simulink model "Lab3Simulink"  (R2024b)
settings: Solver=FixedStepAuto  StartTime=0.0  StopTime=inf  FixedStep=0.01  RelTol=1e-3  EnableMultiTasking=on
libraries: stm32f4xxblockslib x9, simulink x3, stm32g4xxblockslib x3
settings Model: STM32="{\"EncoderBlockForG4\":[{\"ID\":\"Lab3Simulink:156\"},{\"ID\":\"Lab3Simulink:162\"},{\"ID\":\"Lab3Simulink:166\"}],\"DigitalPortRead\":[{\"ID\":\"Lab3Simulink:9\"},{\"ID\":\"Lab3Simulink:11\"},{\"ID\":\"Lab3Simulink:112\"},{\"ID\":\"Lab3Simulink:113\"},{\"ID\":\"Lab3Simulink:119\"},{\"ID\":\"Lab3Simulink:120\"},{\"ID\":\"Lab3Simulink:198\"},{\"ID\":\"Lab3Simulink:199\"},{\"ID\":\"Lab3Simulink:200\"}]}"  Creator=lenovo  LastModifiedBy=lenovo
settings OptimizationCC: DefaultParameterBehavior=Inlined  EnhancedBackFolding=on  PassReuseOutputArgsAs=Individual arguments  ZeroExternalMemoryAtStartup=off  ZeroInternalMemoryAtStartup=off  MaxStackSize=512  OptimizeBlockOrder=speed  DifferentSizesBufferReuse=on  OptimizationCustomize=off  EfficientTunableParamExpr=on
settings DebuggingCC: ParameterTunabilityLossMsg=error
settings HardwareCC: ProdBitPerPointer=32  ProdBitPerSizeT=32  ProdBitPerPtrDiffT=32  ProdLargestAtomicInteger=Long  ProdLargestAtomicFloat=Double  ProdWordSize=32  ProdLongLongMode=on  ProdHWDeviceType=ARM Compatible->ARM Cortex-M
settings SFSimCC: MATLABDynamicMemAlloc=off
settings RTWCC: Description=Embedded Coder  SystemTargetFile=ert.tlc  HardwareBoard=STM32G4xx Based  TemplateMakefile=ert_default_tmf  Toolchain=GNU Tools for ARM Embedded Processors
settings CodeAppCC: ForceParamTrailComments=on  IgnoreCustomStorageClasses=off  OperatorAnnotations=on  SimulinkDataObjDesc=on  SFDataObjDesc=on  InsertBlockDesc=on
settings ERTTargetCC: TargetLangStandard=C99 (ISO)  CodeReplacementLibrary=ARM Cortex-M  ExtModeTransport=3  ExtModeStaticAlloc=on  ExtModeStaticAllocSize=2048  ExtModeMexFile=ext_xcp  ExtModeIntrfLevel=Level2 - Open

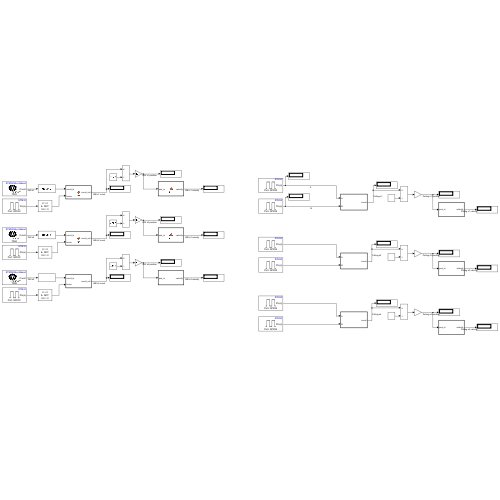
[thumbnail: Simulink's stored preview of the top-level diagram]
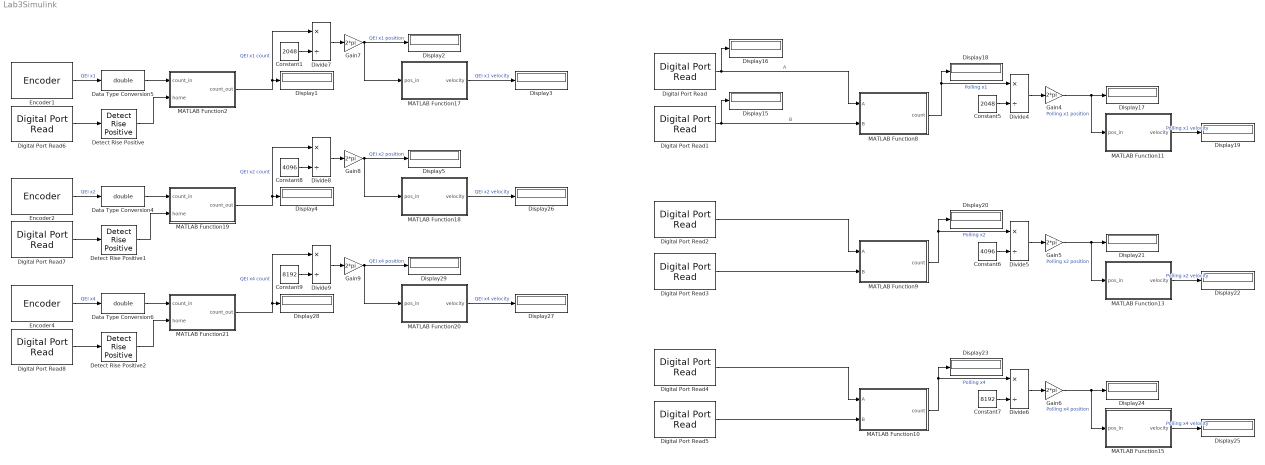
== system Lab3Simulink ==
  Constant1 : Constant  Value=2048
  Constant5 : Constant  Value=2048
  Constant6 : Constant  Value=4096
  Constant7 : Constant  Value=8192
  Constant8 : Constant  Value=4096
  Constant9 : Constant  Value=8192
  Data Type Conversion4 : DataTypeConversion  OutDataTypeStr=double  SaturateOnIntegerOverflow=off  RndMeth=Floor
  Data Type Conversion5 : DataTypeConversion  OutDataTypeStr=double  SaturateOnIntegerOverflow=off  RndMeth=Floor
  Data Type Conversion6 : DataTypeConversion  OutDataTypeStr=double  SaturateOnIntegerOverflow=off  RndMeth=Floor
  Detect Rise Positive : simulink/Logic and Bit Operations/Detect Rise Positive  vinit=0  OutDataTypeStr=boolean
  Detect Rise Positive1 : simulink/Logic and Bit Operations/Detect Rise Positive  vinit=0  OutDataTypeStr=boolean
  Detect Rise Positive2 : simulink/Logic and Bit Operations/Detect Rise Positive  vinit=0  OutDataTypeStr=boolean
  Digital Port Read : stm32f4xxblockslib/Digital Port Read  PortName=GPIOB  PinNumber=[4]  ReadOperation=on  IOAsArray=on  SampleTime=-1  EnableSimPort=off  hoistedMaskSrc=ECSoC/ECSimCodegen/Digital Port Read
      settings: LibrarySourceBlock=stm32g4xxblockslib/Digital Port Read
  Digital Port Read1 : stm32f4xxblockslib/Digital Port Read  PortName=GPIOB  PinNumber=[5]  ReadOperation=on  IOAsArray=on  SampleTime=-1  EnableSimPort=off  hoistedMaskSrc=ECSoC/ECSimCodegen/Digital Port Read
      settings: LibrarySourceBlock=stm32g4xxblockslib/Digital Port Read
  Digital Port Read2 : stm32f4xxblockslib/Digital Port Read  PortName=GPIOB  PinNumber=[4]  ReadOperation=on  IOAsArray=on  SampleTime=-1  EnableSimPort=off  hoistedMaskSrc=ECSoC/ECSimCodegen/Digital Port Read
      settings: LibrarySourceBlock=stm32g4xxblockslib/Digital Port Read
  Digital Port Read3 : stm32f4xxblockslib/Digital Port Read  PortName=GPIOB  PinNumber=[5]  ReadOperation=on  IOAsArray=on  SampleTime=-1  EnableSimPort=off  hoistedMaskSrc=ECSoC/ECSimCodegen/Digital Port Read
      settings: LibrarySourceBlock=stm32g4xxblockslib/Digital Port Read
  Digital Port Read4 : stm32f4xxblockslib/Digital Port Read  PortName=GPIOB  PinNumber=[4]  ReadOperation=on  IOAsArray=on  SampleTime=-1  EnableSimPort=off  hoistedMaskSrc=ECSoC/ECSimCodegen/Digital Port Read
      settings: LibrarySourceBlock=stm32g4xxblockslib/Digital Port Read
  Digital Port Read5 : stm32f4xxblockslib/Digital Port Read  PortName=GPIOB  PinNumber=[5]  ReadOperation=on  IOAsArray=on  SampleTime=-1  EnableSimPort=off  hoistedMaskSrc=ECSoC/ECSimCodegen/Digital Port Read
      settings: LibrarySourceBlock=stm32g4xxblockslib/Digital Port Read
  Digital Port Read6 : stm32f4xxblockslib/Digital Port Read  PortName=GPIOC  PinNumber=[13]  ReadOperation=on  IOAsArray=on  SampleTime=-1  EnableSimPort=off  hoistedMaskSrc=ECSoC/ECSimCodegen/Digital Port Read
      settings: LibrarySourceBlock=stm32g4xxblockslib/Digital Port Read
  Digital Port Read7 : stm32f4xxblockslib/Digital Port Read  PortName=GPIOC  PinNumber=[13]  ReadOperation=on  IOAsArray=on  SampleTime=-1  EnableSimPort=off  hoistedMaskSrc=ECSoC/ECSimCodegen/Digital Port Read
      settings: LibrarySourceBlock=stm32g4xxblockslib/Digital Port Read
  Digital Port Read8 : stm32f4xxblockslib/Digital Port Read  PortName=GPIOC  PinNumber=[13]  ReadOperation=on  IOAsArray=on  SampleTime=-1  EnableSimPort=off  hoistedMaskSrc=ECSoC/ECSimCodegen/Digital Port Read
      settings: LibrarySourceBlock=stm32g4xxblockslib/Digital Port Read
  Display{1..5,15..29} (20 alike) : Display
  Divide{4..9} (6 alike) : Product  Inputs=*/
  Encoder1 : stm32g4xxblockslib/Encoder  TimerModule=TIM3  EnableResetInput=off  OutputCountAfterFirstIndex=off  OutputValidIndex=off  OutputDirection=off  OutputStatus=off  SampleTime=-1
  Encoder2 : stm32g4xxblockslib/Encoder  TimerModule=TIM4  EnableResetInput=off  OutputCountAfterFirstIndex=off  OutputValidIndex=off  OutputDirection=off  OutputStatus=off  SampleTime=-1
  Encoder4 : stm32g4xxblockslib/Encoder  TimerModule=TIM8  EnableResetInput=off  OutputCountAfterFirstIndex=off  OutputValidIndex=off  OutputDirection=off  OutputStatus=off  SampleTime=-1
  Gain{4..9} (6 alike) : Gain  Gain=2*pi
  MATLAB Function10 : MATLAB Function  TreatAsAtomicUnit=on
  MATLAB Function11 : MATLAB Function  TreatAsAtomicUnit=on
  MATLAB Function13 : MATLAB Function  TreatAsAtomicUnit=on
  MATLAB Function15 : MATLAB Function  TreatAsAtomicUnit=on
  MATLAB Function17 : MATLAB Function  TreatAsAtomicUnit=on
  MATLAB Function18 : MATLAB Function  TreatAsAtomicUnit=on
  MATLAB Function19 : MATLAB Function  TreatAsAtomicUnit=on
  MATLAB Function2 : MATLAB Function  TreatAsAtomicUnit=on
  MATLAB Function20 : MATLAB Function  TreatAsAtomicUnit=on
  MATLAB Function21 : MATLAB Function  TreatAsAtomicUnit=on
  MATLAB Function8 : MATLAB Function  TreatAsAtomicUnit=on
  MATLAB Function9 : MATLAB Function  TreatAsAtomicUnit=on
  wires:
  Digital Port Read1/1 -> Display15/1, MATLAB Function8/2(B)  "B"
  Digital Port Read/1 -> MATLAB Function8/1(A), Display16/1  "A"
  MATLAB Function8/1(count) -> Divide4/1, Display18/1  "Polling x1"
  MATLAB Function9/1(count) -> Divide5/1, Display20/1  "Polling x2"
  Digital Port Read3/1 -> MATLAB Function9/2(B)
  Digital Port Read5/1 -> MATLAB Function10/2(B)
  MATLAB Function10/1(count) -> Divide6/1, Display23/1  "Polling x4"
  Digital Port Read4/1 -> MATLAB Function10/1(A)
  Digital Port Read2/1 -> MATLAB Function9/1(A)
  Gain4/1 -> MATLAB Function11/1(pos_in), Display17/1  "Polling x1 position"
  Constant5/1 -> Divide4/2
  MATLAB Function11/1(velocity) -> Display19/1  "Polling x1 velocity"
  Constant6/1 -> Divide5/2
  MATLAB Function13/1(velocity) -> Display22/1  "Polling x2 velocity"
  Gain5/1 -> MATLAB Function13/1(pos_in), Display21/1  "Polling x2 position"
  Constant7/1 -> Divide6/2
  MATLAB Function15/1(velocity) -> Display25/1  "Polling x4 velocity"
  Gain6/1 -> MATLAB Function15/1(pos_in), Display24/1  "Polling x4 position"
  Encoder1/1 -> Data Type Conversion5/1  "QEI x1"
  Data Type Conversion5/1 -> MATLAB Function2/1(count_in)
  MATLAB Function2/1(count_out) -> Divide7/1, Display1/1  "QEI x1 count"
  Encoder2/1 -> Data Type Conversion4/1  "QEI x2"
  Encoder4/1 -> Data Type Conversion6/1  "QEI x4"
  Constant1/1 -> Divide7/2
  Divide7/1 -> Gain7/1
  Gain7/1 -> MATLAB Function17/1(pos_in), Display2/1  "QEI x1 position"
  MATLAB Function17/1(velocity) -> Display3/1  "QEI x1 velocity"
  MATLAB Function18/1(velocity) -> Display26/1  "QEI x2 velocity"
  Gain8/1 -> Display5/1, MATLAB Function18/1(pos_in)  "QEI x2 position"
  Divide8/1 -> Gain8/1
  Constant8/1 -> Divide8/2
  MATLAB Function19/1(count_out) -> Display4/1, Divide8/1  "QEI x2 count"
  Data Type Conversion4/1 -> MATLAB Function19/1(count_in)
  Data Type Conversion6/1 -> MATLAB Function21/1(count_in)
  MATLAB Function21/1(count_out) -> Divide9/1, Display28/1  "QEI x4 count"
  Constant9/1 -> Divide9/2
  Divide9/1 -> Gain9/1
  Gain9/1 -> MATLAB Function20/1(pos_in), Display29/1  "QEI x4 position"
  MATLAB Function20/1(velocity) -> Display27/1  "QEI x4 velocity"
  Divide4/1 -> Gain4/1
  Divide5/1 -> Gain5/1
  Divide6/1 -> Gain6/1
  Digital Port Read6/1 -> Detect Rise Positive/1
  Detect Rise Positive/1 -> MATLAB Function2/2(home)
  Digital Port Read7/1 -> Detect Rise Positive1/1
  Detect Rise Positive1/1 -> MATLAB Function19/2(home)
  Digital Port Read8/1 -> Detect Rise Positive2/1
  Detect Rise Positive2/1 -> MATLAB Function21/2(home)

== matlab function Lab3Simulink/MATLAB Function17 ==
  data: pos_in input; velocity output
function velocity = fcn(pos_in)
persistent pev_pos;
if isempty(pev_pos)
    pev_pos = 0;
end

velocity = (pos_in - pev_pos) / 0.01;
pev_pos = pos_in;

== matlab function Lab3Simulink/MATLAB Function8 ==
  data: A input; count output; B input
function count = quadratureDecodeX1(A, B)
    persistent prevA prevcount;
    if isempty(prevA)
        prevA = A;
        prevcount = 0;
    end

    if prevA == 0 && A == 1
        if B == 1
            prevcount = prevcount + 1;  % Forward direction
        else
            prevcount = prevcount - 1;  % Reverse direction
        end
    end
    prevA = A;
    count = prevcount;
end

== matlab function Lab3Simulink/MATLAB Function9 ==
  data: A input; count output; B input
function count = quadratureDecodeX2(A, B)
    persistent prevA prevcount;
    if isempty(prevA)
        prevA = A;
        prevcount = 0;
    end
    
    if prevA ~= A
        if A == 1  % Rising edge of A
            if B == 1
                prevcount = prevcount + 1;  % Forward direction
            else
                prevcount = prevcount - 1;  % Reverse direction
            end
        else  % Falling edge of A
            if B == 0
                prevcount = prevcount + 1;  % Forward direction
            else
                prevcount = prevcount - 1;  % Reverse direction
            end
        end
    end
    prevA = A;
    count = prevcount;
end

== matlab function Lab3Simulink/MATLAB Function10 ==
  data: A input; count output; B input
function count = quadratureDecode(A, B)
persistent prevA prevB prevcount;
if isempty(prevA)
    prevA = A;
    prevB = B;
    prevcount = 0;
end
    
    if prevA == 0 && A == 1      % Rising edge on A
        if B == 0
            prevcount = prevcount + 1;   % Forward direction
        else
            prevcount = prevcount - 1;   % Reverse direction
        end
    elseif prevA == 1 && A == 0  % Falling edge on A
        if B == 1
            prevcount = prevcount + 1;   % Forward direction
        else
            prevcount = prevcount - 1;   % Reverse direction
        end
    elseif prevB == 0 && B == 1  % Rising edge on B
        if A == 1
            prevcount = prevcount + 1;   % Forward direction
        else
            prevcount = prevcount - 1;   % Reverse direction
        end
    elseif prevB == 1 && B == 0  % Falling edge on B
        if A == 0
            prevcount = prevcount + 1;   % Forward direction
        else
            prevcount = prevcount - 1;   % Reverse direction
        end
    end
    prevA = A;
    prevB = B;
    count = prevcount * (-1);
end

== matlab function Lab3Simulink/MATLAB Function11 ==
  data: pos_in input; velocity output
function velocity = fcn(pos_in)
persistent pev_pos;
if isempty(pev_pos)
    pev_pos = 0;
end

velocity = (pos_in - pev_pos) / 0.01;
pev_pos = pos_in;

== matlab function Lab3Simulink/MATLAB Function13 ==
  data: pos_in input; velocity output
function velocity = fcn(pos_in)
persistent pev_pos;
if isempty(pev_pos)
    pev_pos = 0;
end

velocity = (pos_in - pev_pos) / 0.01;
pev_pos = pos_in;

== matlab function Lab3Simulink/MATLAB Function15 ==
  data: pos_in input; velocity output
function velocity = fcn(pos_in)
persistent pev_pos;
if isempty(pev_pos)
    pev_pos = 0;
end

velocity = (pos_in - pev_pos) / 0.01;
pev_pos = pos_in;

== matlab function Lab3Simulink/MATLAB Function18 ==
  data: pos_in input; velocity output
function velocity = fcn(pos_in)
persistent pev_pos;
if isempty(pev_pos)
    pev_pos = 0;
end

velocity = (pos_in - pev_pos) / 0.01;
pev_pos = pos_in;

== matlab function Lab3Simulink/MATLAB Function19 ==
  data: count_in input; count_out output; home input
function count_out = fcn(count_in, home)
    % Define persistent variables
    persistent count;
    persistent n;
    persistent temp_count;

    if home == 1
        temp_count = count_in;
    end

    % Initialize the persistent variables if empty
    if isempty(count)
        count = 0;
    end
    if isempty(n)
        n = 0;
    end
    if isempty(temp_count)
        temp_count = 0;
    end

    cr = 49152;
    cr2 = cr / 2;
    % Calculate the difference
    delta = count_in - n;

    % Detect overflow or underflow and adjust count accordingly
    if delta <= -cr2
        count = count + cr;
    elseif delta >= cr2
        count = count - cr;
    end

    % Update the previous value of count_in
    n = count_in;

    % Output the adjusted count
   count_out = count + count_in - temp_count;
 
end

== matlab function Lab3Simulink/MATLAB Function2 ==
  data: count_in input; count_out output; home input
function count_out = fcn(count_in, home)
    persistent count;
    persistent n;
    persistent temp_count;
    if home == 1
        temp_count = count_in;
    end
    if isempty(count)
        count = 0;
    end
    if isempty(n)
        n = 0;
    end
    if isempty(temp_count)
        temp_count = 0;
    end
    cr = 49152;
    cr2 = cr / 2;
    delta = count_in - n;
    if delta <= -cr2
        count = count + cr;
    elseif delta >= cr2
        count = count - cr;
    end
    n = count_in;
    count_out = count + count_in - temp_count;
end

== matlab function Lab3Simulink/MATLAB Function20 ==
  data: pos_in input; velocity output
function velocity = fcn(pos_in)
persistent pev_pos;
if isempty(pev_pos)
    pev_pos = 0;
end

velocity = (pos_in - pev_pos) / 0.01;
pev_pos = pos_in;

== matlab function Lab3Simulink/MATLAB Function21 ==
  data: count_in input; count_out output; home input
function count_out = fcn(count_in, home)
    % Define persistent variables
    persistent count;
    persistent n;
    persistent temp_count;

    if home == 1
        temp_count = count_in;
    end

    % Initialize the persistent variables if empty
    if isempty(count)
        count = 0;
    end
    if isempty(n)
        n = 0;
    end
    if isempty(temp_count)
        temp_count = 0;
    end

    cr = 49152;
    cr2 = cr / 2;
    % Calculate the difference
    delta = count_in - n;

    % Detect overflow or underflow and adjust count accordingly
    if delta <= -cr2
        count = count + cr;
    elseif delta >= cr2
        count = count - cr;
    end

    % Update the previous value of count_in
    n = count_in;

    % Output the adjusted count
   count_out = count + count_in - temp_count;
 
end
